simulink library "fminconTest"  (R2018b)
settings: Solver=VariableStepAuto  StartTime=0.0  StopTime=10.0  RelTol=1e-3
settings Model: Creator=Ayaz  LastModifiedBy=Ayaz

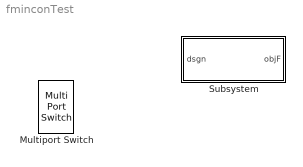
== system fminconTest ==
  Multiport Switch : MultiPortSwitch
  Subsystem : Subsystem

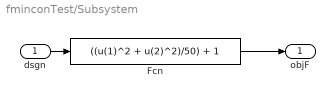
== system fminconTest/Subsystem ==
  dsgn : Inport
  Fcn : Fcn  Expr=((u(1)^2 + u(2)^2)/50) + 1
  objF : Outport
  wires:
  dsgn/1 -> Fcn/1
  Fcn/1 -> objF/1
